simulink model "uz_resolver_pl_interface"  (R2021a)
settings: Solver=FixedStepDiscrete  StartTime=0.0  StopTime=3/f_mech*resolver_polepairs*2  RelTol=1e-3
values from neighbouring files (symbols this model uses):
  bitToRpsFactor_16bit = rps_max_16bit/(2^(16-1))    (= 0.00381469726562)    [uz_resolver_mech_revolution_calc_init.m]
  f_mech = 500    [uz_resolver_mech_revolution_calc_init.m]
  machine_polepairs = 5    [uz_resolver_mech_revolution_calc_init.m]
  resolver_polepairs = 3    [uz_resolver_mech_revolution_calc_init.m]
  t_ADC = 1/f_ADC    (= 1e-05)    [uz_resolver_mech_revolution_calc_init.m]
undefined symbols (not defined in the file or in its folder): theta_m_offset
libraries: simulink x1
settings Model: DataTypeOverride=Off  Creator=micha  LastModifiedBy=micha
settings SolverCC: AlgebraicLoopSolver=TrustRegion
settings DataIOCC: LimitDataPoints=on  SaveOutput=off  SaveTime=off
settings OptimizationCC: BlockReduction=off  ConditionallyExecuteInputs=off  DefaultParameterBehavior=Inlined  LifeSpan=inf
settings DebuggingCC: AlgebraicLoopMsg=error  SingleTaskRateTransMsg=error  AllowSymbolicDim=off  StrictBusMsg=ErrorOnBusTreatedAsVector  SFUnexpectedBacktrackingDiag=warning  SFNoUnconditionalDefaultTransitionDiag=warning  SFExecutionAtInitializationDiag=none  SFMachineParentedDataDiag=warning  ArithmeticOperatorsInVariantConditions=warning
settings HardwareCC: ProdBitPerPointer=32  ProdBitPerSizeT=32  ProdBitPerPtrDiffT=32  ProdLargestAtomicFloat=None  ProdIntDivRoundTo=Undefined  ProdEndianess=Unspecified  ProdWordSize=32  ProdHWDeviceType=ASIC/FPGA->ASIC/FPGA  ProdEqTarget=off
settings SFSimCC: SimUseLocalCustomCode=off  CustomCodeUndefinedFunction=UseInterfaceOnly
settings RTWCC: RTWUseLocalCustomCode=off
settings CodeAppCC: StateflowObjectComments=on
settings GRTTargetCC: TargetLangStandard=C89/C90 (ANSI)
settings ConfigComp: CovScope=ReferencedModels  CovMetricSettings=dw  CovSaveCumulativeToWorkspaceVar=on  CovSaveSingleToWorkspaceVar=on  CovExternalEMLEnable=off  CovSFcnEnable=off

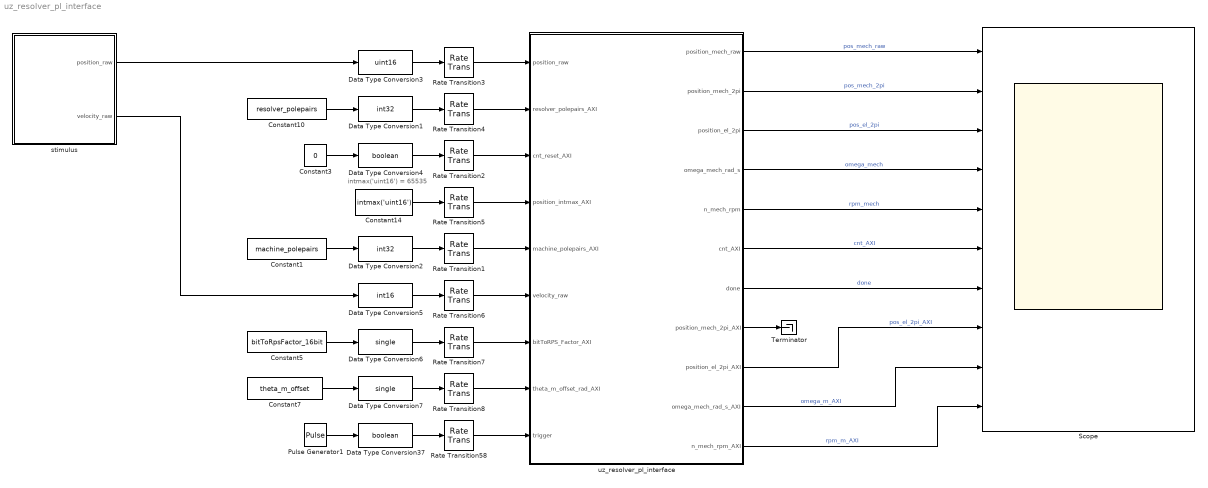
== system uz_resolver_pl_interface ==
  note: intmax('uint16') = 65535
  Constant1 : Constant  Value=machine_polepairs
  Constant10 : Constant  Value=resolver_polepairs
  Constant14 : Constant  Value=intmax('uint16')  OutDataTypeStr=int32  SampleTime=-1
  Constant3 : Constant  Value=0
  Constant5 : Constant  Value=bitToRpsFactor_16bit  SampleTime=-1
  Constant7 : Constant  Value=theta_m_offset  OutDataTypeStr=single  SampleTime=-1
  Data Type Conversion1 : DataTypeConversion  OutDataTypeStr=int32
  Data Type Conversion2 : DataTypeConversion  OutDataTypeStr=int32
  Data Type Conversion3 : DataTypeConversion  OutDataTypeStr=uint16
  Data Type Conversion37 : DataTypeConversion  OutDataTypeStr=boolean
  Data Type Conversion4 : DataTypeConversion  OutDataTypeStr=boolean
  Data Type Conversion5 : DataTypeConversion  OutDataTypeStr=int16
  Data Type Conversion6 : DataTypeConversion  OutDataTypeStr=single
  Data Type Conversion7 : DataTypeConversion  OutDataTypeStr=single
  Pulse Generator1 : DiscretePulseGenerator  PulseType=Time based  Period=t_ADC  PulseWidth=5
  Rate Transition{1..8,58} (9 alike) : RateTransition  OutPortSampleTime=t_clock
  Scope : Scope  NumInputPorts=10
  Terminator : Terminator
  stimulus : Subsystem
  uz_resolver_pl_interface : Subsystem  TreatAsAtomicUnit=on
  wires:
  Rate Transition58/1 -> uz_resolver_pl_interface/9(trigger)
  Data Type Conversion4/1 -> Rate Transition2/1
  Data Type Conversion37/1 -> Rate Transition58/1
  Pulse Generator1/1 -> Data Type Conversion37/1
  Rate Transition4/1 -> uz_resolver_pl_interface/2(resolver_polepairs_AXI)
  Rate Transition3/1 -> uz_resolver_pl_interface/1(position_raw)
  Rate Transition2/1 -> uz_resolver_pl_interface/3(cnt_reset_AXI)
  Constant14/1 -> Rate Transition5/1
  Rate Transition5/1 -> uz_resolver_pl_interface/4(position_intmax_AXI)
  Data Type Conversion3/1 -> Rate Transition3/1
  Constant10/1 -> Data Type Conversion1/1
  Data Type Conversion1/1 -> Rate Transition4/1
  uz_resolver_pl_interface/1(position_mech_raw) -> Scope/1  "pos_mech_raw"
  uz_resolver_pl_interface/2(position_mech_2pi) -> Scope/2  "pos_mech_2pi"
  uz_resolver_pl_interface/6(cnt_AXI) -> Scope/6  "cnt_AXI"
  uz_resolver_pl_interface/7(done) -> Scope/7  "done"
  stimulus/1(position_raw) -> Data Type Conversion3/1
  Data Type Conversion2/1 -> Rate Transition1/1
  Constant1/1 -> Data Type Conversion2/1
  Rate Transition1/1 -> uz_resolver_pl_interface/5(machine_polepairs_AXI)
  uz_resolver_pl_interface/3(position_el_2pi) -> Scope/3  "pos_el_2pi"
  Data Type Conversion5/1 -> Rate Transition6/1
  Rate Transition6/1 -> uz_resolver_pl_interface/6(velocity_raw)
  stimulus/2(velocity_raw) -> Data Type Conversion5/1
  Rate Transition7/1 -> uz_resolver_pl_interface/7(bitToRPS_Factor_AXI)
  Data Type Conversion6/1 -> Rate Transition7/1
  Constant5/1 -> Data Type Conversion6/1
  uz_resolver_pl_interface/4(omega_mech_rad_s) -> Scope/4  "omega_mech"
  uz_resolver_pl_interface/5(n_mech_rpm) -> Scope/5  "rpm_mech"
  uz_resolver_pl_interface/9(position_el_2pi_AXI) -> Scope/8  "pos_el_2pi_AXI"
  uz_resolver_pl_interface/8(position_mech_2pi_AXI) -> Terminator/1
  uz_resolver_pl_interface/10(omega_mech_rad_s_AXI) -> Scope/9  "omega_m_AXI"
  uz_resolver_pl_interface/11(n_mech_rpm_AXI) -> Scope/10  "rpm_m_AXI"
  Constant3/1 -> Data Type Conversion4/1
  Constant7/1 -> Data Type Conversion7/1
  Rate Transition8/1 -> uz_resolver_pl_interface/8(theta_m_offset_rad_AXI)
  Data Type Conversion7/1 -> Rate Transition8/1

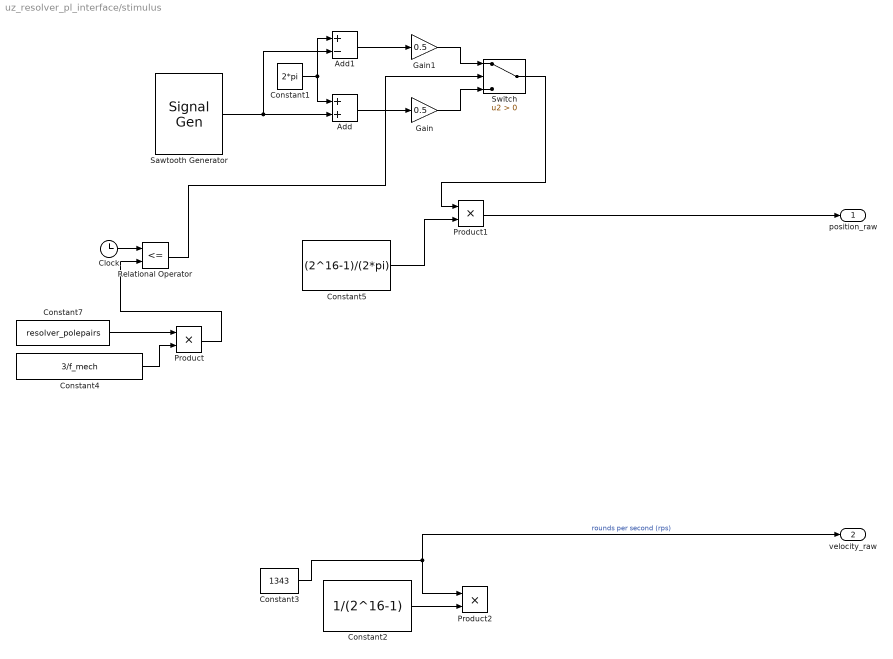
== system uz_resolver_pl_interface/stimulus ==
  Add : Sum
  Add1 : Sum  Inputs=+-
  Clock : Clock
  Constant1 : Constant  Value=2*pi
  Constant2 : Constant  Value=1/(2^16-1)
  Constant3 : Constant  Value=1343  SampleTime=-1
  Constant4 : Constant  Value=3/f_mech
  Constant5 : Constant  Value=(2^16-1)/(2*pi)
  Constant7 : Constant  Value=resolver_polepairs
  Gain : Gain  Gain=0.5
  Gain1 : Gain  Gain=0.5
  Product : Product
  Product1 : Product
  Product2 : Product
  Relational Operator : RelationalOperator  Operator=<=  OutDataTypeStr=boolean  RndMeth=Simplest
  Sawtooth Generator : SignalGenerator  WaveForm=sawtooth  Amplitude=2*pi  Frequency=2*pi*f_mech  Units=rad/sec
  Switch : Switch  Criteria=u2 > Threshold
  position_raw : Outport
  velocity_raw : Outport  Port=2
  wires:
  Sawtooth Generator/1 -> Add1/2, Add/2
  Constant4/1 -> Product/2
  Clock/1 -> Relational Operator/1
  Gain/1 -> Switch/3
  Constant5/1 -> Product1/2
  Product/1 -> Relational Operator/2
  Add1/1 -> Gain1/1
  Gain1/1 -> Switch/1
  Constant1/1 -> Add/1, Add1/1
  Add/1 -> Gain/1
  Constant7/1 -> Product/1
  Relational Operator/1 -> Switch/2
  Product1/1 -> position_raw/1
  Constant2/1 -> Product2/2
  Constant3/1 -> velocity_raw/1, Product2/1  "rounds per second (rps)"
  Switch/1 -> Product1/1

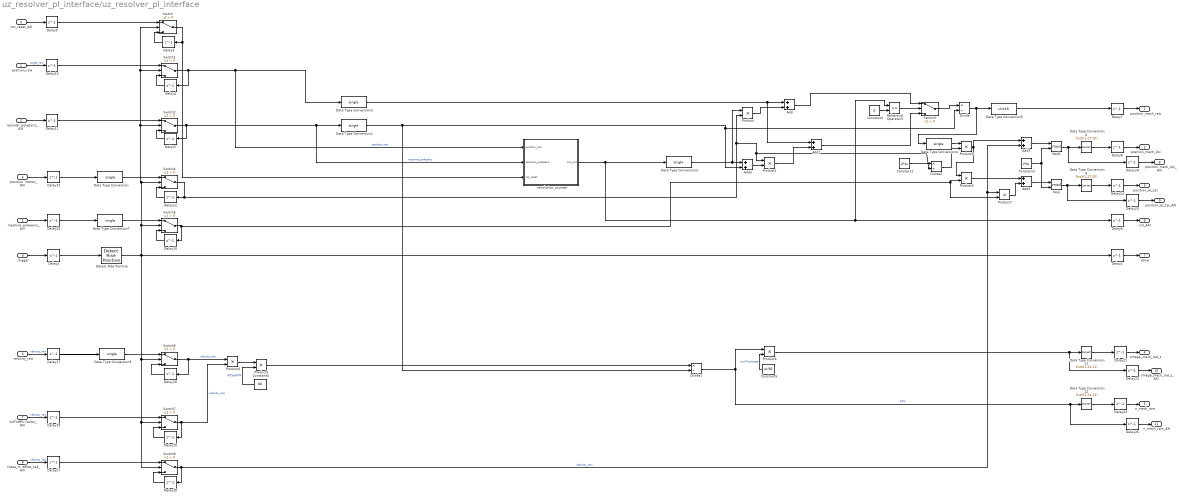
== system uz_resolver_pl_interface/uz_resolver_pl_interface ==
  position_raw : Inport
  resolver_polepairs_AXI : Inport  Port=2
  cnt_reset_AXI : Inport  Port=3
  position_intmax_AXI : Inport  Port=4
  machine_polepairs_AXI : Inport  Port=5
  velocity_raw : Inport  Port=6
  bitToRPS_Factor_AXI : Inport  Port=7
  theta_m_offset_rad_AXI : Inport  Port=8
  trigger : Inport  Port=9
  Add{,1..3,5} (5 alike) : Sum
  Constant1 : Constant  Value=2*pi  OutDataTypeStr=single  SampleTime=-1
  Constant2 : Constant  Value=0  OutDataTypeStr=int16  SampleTime=-1
  Constant3 : Constant  Value=2*pi  OutDataTypeStr=single  SampleTime=-1
  Constant4 : Constant  Value=60  OutDataTypeStr=single  SampleTime=-1
  Constant5 : Constant  Value=pi/30  OutDataTypeStr=single  SampleTime=-1
  Data Type Conversion{,1..4,7,9} (7 alike) : DataTypeConversion  OutDataTypeStr=single
  Data Type Conversion11 : DataTypeConversion  OutDataTypeStr=fixdt(1,24,11)
  Data Type Conversion12 : DataTypeConversion  OutDataTypeStr=fixdt(1,24,11)
  Data Type Conversion5 : DataTypeConversion  OutDataTypeStr=uint16
  Data Type Conversion6 : DataTypeConversion  OutDataTypeStr=fixdt(1,27,20)
  Data Type Conversion8 : DataTypeConversion  OutDataTypeStr=fixdt(1,27,20)
  Delay{1..3,6..11,13..28} (25 alike) : Delay  DelayLength=1
  Delay12 : Delay  DelayLength=1  InitialCondition=intmax('uint16')
  Delay4 : Delay  DelayLength=1  InitialCondition=0
  Delay5 : Delay  DelayLength=1  InitialCondition=resolver_polepairs
  Detect Rise Positive : simulink/Logic and Bit Operations/Detect Rise Positive  vinit=0  OutDataTypeStr=boolean
  Divide : Product  Inputs=*/  RndMeth=Simplest  SaturateOnIntegerOverflow=on
  Divide1 : Product  Inputs=*/
  Divide2 : Product  Inputs=*/  RndMeth=Simplest  SaturateOnIntegerOverflow=on
  Mod : Math  Operator=mod  OutputSignalType=real  SaturateOnIntegerOverflow=on
  Mod1 : Math  Operator=mod  OutputSignalType=real  SaturateOnIntegerOverflow=on
  Product{,1..7} (8 alike) : Product
  Relational Operator5 : RelationalOperator  OutDataTypeStr=boolean  RndMeth=Simplest
  Switch{,1..8} (9 alike) : Switch  Criteria=u2 > Threshold
  revolution_counter : MATLAB Function  TreatAsAtomicUnit=on
  position_mech_raw : Outport  VectorParamsAs1DForOutWhenUnconnected=off
  position_mech_2pi : Outport  Port=2  VectorParamsAs1DForOutWhenUnconnected=off
  position_el_2pi : Outport  Port=3  VectorParamsAs1DForOutWhenUnconnected=off
  omega_mech_rad_s : Outport  Port=4  VectorParamsAs1DForOutWhenUnconnected=off
  n_mech_rpm : Outport  Port=5  VectorParamsAs1DForOutWhenUnconnected=off
  cnt_AXI : Outport  Port=6  VectorParamsAs1DForOutWhenUnconnected=off
  done : Outport  Port=7  VectorParamsAs1DForOutWhenUnconnected=off
  position_mech_2pi_AXI : Outport  Port=8  VectorParamsAs1DForOutWhenUnconnected=off
  position_el_2pi_AXI : Outport  Port=9  VectorParamsAs1DForOutWhenUnconnected=off
  omega_mech_rad_s_AXI : Outport  Port=10  VectorParamsAs1DForOutWhenUnconnected=off
  n_mech_rpm_AXI : Outport  Port=11  VectorParamsAs1DForOutWhenUnconnected=off
  wires:
  Switch2/1 -> Delay5/1, revolution_counter/2(resolver_polepairs), Data Type Conversion1/1  "resolver_polepairs"
  Switch1/1 -> Delay4/1, revolution_counter/1(position_raw), Data Type Conversion2/1  "position_raw"
  Switch/1 -> Delay3/1, revolution_counter/3(cnt_reset)
  Delay1/1 -> Detect Rise Positive/1
  trigger/1 -> Delay1/1
  Delay2/1 -> done/1
  cnt_reset_AXI/1 -> Delay9/1
  position_raw/1 -> Delay10/1  "angle_raw"
  resolver_polepairs_AXI/1 -> Delay11/1
  Delay3/1 -> Switch/3
  Delay4/1 -> Switch1/3
  Delay5/1 -> Switch2/3
  Delay6/1 -> cnt_AXI/1
  Delay7/1 -> position_mech_raw/1
  Delay8/1 -> position_mech_2pi/1
  Constant2/1 -> Relational Operator5/2
  Relational Operator5/1 -> Switch3/2
  Switch4/1 -> Product/2, Divide2/2, Product1/1, Delay12/1
  Product/1 -> Add/2
  Switch3/1 -> Divide/1
  Divide/1 -> Data Type Conversion5/1, Data Type Conversion4/1
  Add/1 -> Switch3/1
  Add5/1 -> Product1/2
  Product1/1 -> Add1/2
  Add1/1 -> Switch3/3
  revolution_counter/1(cnt_out) -> Relational Operator5/1, Delay6/1, Data Type Conversion3/1
  Delay12/1 -> Switch4/3
  position_intmax_AXI/1 -> Delay13/1
  Delay13/1 -> Data Type Conversion/1
  Data Type Conversion/1 -> Switch4/1
  Product2/1 -> Add3/1, Product3/1
  Constant1/1 -> Divide2/1
  Divide2/1 -> Product2/2
  Delay11/1 -> Switch2/1
  Delay10/1 -> Switch1/1
  Delay9/1 -> Switch/1
  Data Type Conversion1/1 -> Divide1/2, Add5/2, Divide/2
  Data Type Conversion2/1 -> Add1/1, Add/1
  Data Type Conversion3/1 -> Add5/1, Product/1
  Data Type Conversion4/1 -> Product2/1
  Data Type Conversion5/1 -> Delay7/1
  Data Type Conversion6/1 -> Delay8/1
  Switch5/1 -> Product7/2, Product3/2, Delay16/1
  Delay14/1 -> position_el_2pi/1
  machine_polepairs_AXI/1 -> Delay15/1
  Delay15/1 -> Data Type Conversion7/1
  Data Type Conversion7/1 -> Switch5/1
  Delay16/1 -> Switch5/3
  Mod/1 -> Delay23/1, Data Type Conversion8/1
  Data Type Conversion8/1 -> Delay14/1
  Product3/1 -> Add2/1
  Constant3/1 -> Mod/2, Mod1/2
  Switch6/1 -> Product4/1, Delay18/1  "velocity_raw"
  Delay17/1 -> Data Type Conversion9/1
  Delay18/1 -> Switch6/3
  velocity_raw/1 -> Delay17/1  "velocity_raw"
  Data Type Conversion9/1 -> Switch6/1
  Product4/1 -> Product5/1
  bitToRPS_Factor_AXI/1 -> Delay19/1  "velocity_raw"
  Delay20/1 -> Switch7/3
  Delay19/1 -> Switch7/1
  Switch7/1 -> Delay20/1, Product4/2  "velocity_raw"
  Constant4/1 -> Product5/2  "RPStoRPM"
  Product5/1 -> Divide1/1
  Divide1/1 -> Delay26/1, Data Type Conversion12/1, Product6/1  "RPM"
  Constant5/1 -> Product6/2  "rpmToomega"
  Product6/1 -> Delay25/1, Data Type Conversion11/1
  Delay21/1 -> omega_mech_rad_s/1
  Data Type Conversion11/1 -> Delay21/1
  Delay22/1 -> n_mech_rpm/1
  Data Type Conversion12/1 -> Delay22/1
  Delay23/1 -> position_el_2pi_AXI/1
  Delay24/1 -> position_mech_2pi_AXI/1
  Delay25/1 -> omega_mech_rad_s_AXI/1
  Delay26/1 -> n_mech_rpm_AXI/1
  Add2/1 -> Mod/1
  Add3/1 -> Mod1/1
  Mod1/1 -> Delay24/1, Data Type Conversion6/1
  Product7/1 -> Add2/2
  Switch8/1 -> Product7/1, Add3/2, Delay28/1  "velocity_raw"
  Delay27/1 -> Switch8/1
  theta_m_offset_rad_AXI/1 -> Delay27/1  "velocity_raw"
  Detect Rise Positive/1 -> Switch8/2, Switch7/2, Switch6/2, Switch5/2, Switch2/2, Switch/2, Switch1/2, Switch4/2, Delay2/1
  Delay28/1 -> Switch8/3

== matlab function uz_resolver_pl_interface/revolution_counter ==
  settings: fimath=fimath('RoundingMethod', 'Floor','OverflowAction', 'Wrap','ProductMode', 'FullPrecision', 'SumMode', 'FullPrecision')
  data: position_raw input; cnt_out output; resolver_polepairs input; cnt_reset input
function cnt_out  = fcn(position_raw, resolver_polepairs, cnt_reset)
%#codegen
persistent angle_mech_old;
if isempty(angle_mech_old)
    angle_mech_old = int32(0);
end

persistent cnt;
if isempty(cnt)
    cnt = int32(0);
end

if ((angle_mech_old-int32(position_raw)) > int32(60000))
    cnt = cnt+1;
elseif ((angle_mech_old-int32(position_raw)) < int32(-60000))
    cnt = cnt-1;
end

if (cnt > (resolver_polepairs-1) || cnt < -(resolver_polepairs-1))
    cnt = int32(0);
end

if (cnt_reset == true)
    cnt = int32(0);
end

angle_mech_old = int32(position_raw);
cnt_out = cnt;
end
